simulink model "simulari"  (R2023a)
settings: Solver=VariableStepAuto  StartTime=0.0  StopTime=1  FixedStep=1e-5  RelTol=1e-3
values from neighbouring files (symbols this model uses):
  Bf = 3.35*10^(-4)    (= 0.000335)    [AC.m]    (also in BC.m; D.m; EF.m)
  F = inv(C*inv(-A+B*K)*B)    [EF.m]
  J = 7*10^(-4)    (= 0.0007)    [AC.m]    (also in BC.m; D.m; EF.m)
  K = acker(A,B,[p1, p1,p1])    [EF.m]
  Ke = 0.296    [AC.m]    (also in BC.m; D.m; EF.m)
  KPWM = 38.46    [AC.m]    (also in BC.m; D.m; EF.m)
  Kt = 0.294    [AC.m]    (also in BC.m; D.m; EF.m)
  L = series(Hvths,Hc1)    [AC.m]    (also in BC.m; EF.m = acker(A', C', [-899.132, -899.132, -899.132])')
  La = 10^(-3)    (= 0.001)    [AC.m]    (also in BC.m; D.m; EF.m)
  Ra = 0.92    [AC.m]    (also in BC.m; D.m; EF.m)
  Te = 4/3*1e-4    (= 0.000133333333333)    [D.m]    (also in EF.m)
settings Model: Creator=ghisa  LastModifiedBy=ghisa

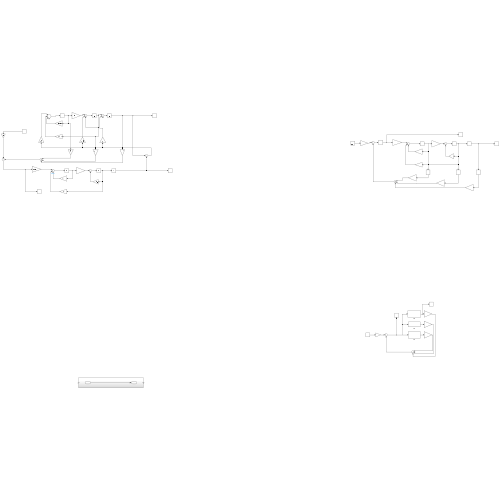
[thumbnail: Simulink's stored preview of the top-level diagram]
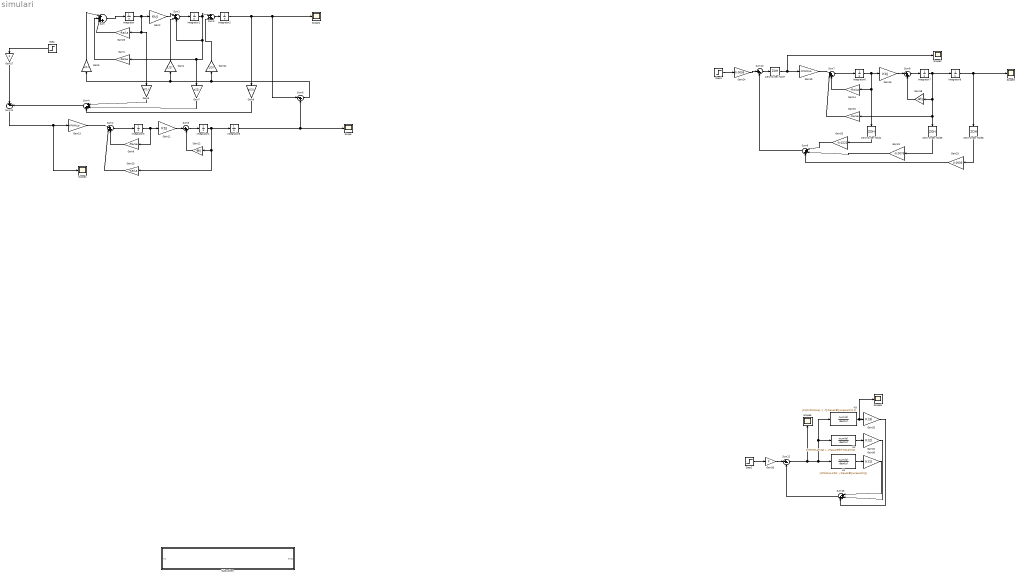
== system simulari ==
  Gain1 : Gain  Gain=-Ke/La
  Gain10 : Gain  Gain=-Ke/La
  Gain11 : Gain  Gain=Kt/J
  Gain12 : Gain  Gain=-Bf/J
  Gain13 : Gain  Gain=KPWM/La
  Gain14 : Gain  Gain=-Ra/La
  Gain15 : Gain  Gain=-Ke/La
  Gain16 : Gain  Gain=Kt/J
  Gain17 : Gain  Gain=F
  Gain18 : Gain  Gain=-Bf/J
  Gain19 : Gain  Gain=KPWM/La
  Gain2 : Gain  Gain=Kt/J
  Gain20 : Gain  Gain=-0.0222
  Gain21 : Gain  Gain=-0.0076
  Gain22 : Gain  Gain=L(3)
  Gain23 : Gain  Gain=0.0006
  Gain24 : Gain  Gain=0.0006
  Gain25 : Gain  Gain=-Ra/La
  Gain30 : Gain  Gain=K(1)
  Gain31 : Gain  Gain=K(2)
  Gain32 : Gain  Gain=K(3)
  Gain33 : Gain  Gain=F
  Gain4 : Gain  Gain=L(2)
  Gain5 : Gain  Gain=L(1)
  Gain6 : Gain  Gain=K(1)
  Gain7 : Gain  Gain=K(2)
  Gain8 : Gain  Gain=K(3)
  Gain9 : Gain  Gain=-Ra/La
  H1 : TransferFcn  Numerator=[KPWM/La KPWM/La*Bf/J]  Denominator=[1 Ra/La+Bf/J Ra/La*Bf/J+Ke/La*Kt/J]
  H2 : TransferFcn  Numerator=[KPWM/La*Kt/J]  Denominator=[1 Ra/La+Bf/J Ra/La*Bf/J+Ke/La*Kt/J]
  H3 : TransferFcn  Numerator=[Kt/J*KPWM/La]  Denominator=[1 Ra/La+Bf/J Ra/La*Bf/J+Ke/La*Kt/J 0]
  Integrator{,1..8} (9 alike) : Integrator
  Scope{,1..6} (7 alike) : Scope
  Step : Step  Time=0  After=100  SampleTime=0
  Step1 : Step  Time=0  After=100  SampleTime=0
  Step2 : Step  Time=0  After=100  SampleTime=0
  Subsystem : Subsystem
  Sum : Sum  Inputs=|++++
  Sum{1..2,4,7,9,15} (6 alike) : Sum  Inputs=|+++
  Sum10 : Sum  Inputs=|+-
  Sum11 : Sum  Inputs=|+-
  Sum12 : Sum  Inputs=|+-
  Sum3 : Sum  Inputs=|++-
  Sum5 : Sum  Inputs=|++
  Sum6 : Sum  Inputs=|-+
  Sum8 : Sum  Inputs=|++
  Zero-Order Hold{4..7} (4 alike) : ZeroOrderHold  SampleTime=Te
  wires:
  Sum1/1 -> Integrator1/1
  Sum/1 -> Integrator/1
  Integrator/1 -> Gain2/1, Gain25/1, Gain6/1
  Gain25/1 -> Sum/3
  Gain1/1 -> Sum/2
  Gain2/1 -> Sum1/1
  Integrator2/1 -> Scope1/1, Sum6/1, Gain8/1
  Gain9/1 -> Sum2/3
  Integrator3/1 -> Gain11/1, Gain9/1
  Integrator4/1 -> Integrator5/1, Gain10/1, Gain12/1
  Gain13/1 -> Sum2/1
  Sum5/1 -> Integrator4/1
  Sum2/1 -> Integrator3/1
  Gain12/1 -> Sum5/2
  Gain10/1 -> Sum2/2
  Gain11/1 -> Sum5/1
  Sum7/1 -> Integrator6/1
  Integrator6/1 -> Gain16/1, Zero-Order Hold4/1, Gain14/1
  Zero-Order Hold6/1 -> Gain23/1
  Gain14/1 -> Sum7/3
  Integrator8/1 -> Scope3/1, Zero-Order Hold6/1
  Gain19/1 -> Sum7/1
  Gain21/1 -> Sum9/2
  Gain20/1 -> Sum9/1
  Zero-Order Hold4/1 -> Gain20/1
  Zero-Order Hold7/1 -> Scope2/1, Gain19/1
  Gain23/1 -> Sum9/3
  Step1/1 -> Gain24/1
  Gain18/1 -> Sum8/2
  Zero-Order Hold5/1 -> Gain21/1
  Gain24/1 -> Sum10/1
  Integrator7/1 -> Integrator8/1, Gain15/1, Zero-Order Hold5/1, Gain18/1
  Sum8/1 -> Integrator7/1
  Gain16/1 -> Sum8/1
  Gain15/1 -> Sum7/2
  Sum9/1 -> Sum10/2
  Sum6/1 -> Gain22/1, Gain5/1, Gain4/1
  Gain5/1 -> Sum/1
  Gain17/1 -> Sum11/1
  Step/1 -> Gain17/1
  Integrator5/1 -> Sum6/2, Scope/1
  Sum11/1 -> Scope4/1, Gain13/1
  Sum3/1 -> Integrator2/1
  Gain22/1 -> Sum3/2
  Integrator1/1 -> Sum3/1, Sum1/3, Gain1/1, Gain7/1
  Gain4/1 -> Sum1/2
  Sum10/1 -> Zero-Order Hold7/1
  Sum15/1 -> Sum12/2
  Gain33/1 -> Sum12/1
  H2/1 -> Gain31/1
  Step2/1 -> Gain33/1
  H1/1 -> Gain30/1
  H3/1 -> Scope6/1, Gain32/1
  Sum12/1 -> H1/1, H3/1, H2/1, Scope5/1
  Gain32/1 -> Sum15/3
  Gain31/1 -> Sum15/2
  Gain30/1 -> Sum15/1
  Gain6/1 -> Sum4/1
  Gain7/1 -> Sum4/2
  Gain8/1 -> Sum4/3
  Sum4/1 -> Sum11/2

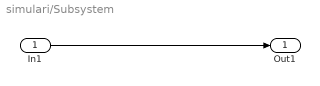
== system simulari/Subsystem ==
  In1 : Inport
  Out1 : Outport
  wires:
  In1/1 -> Out1/1
